simulink model "c172pJSBSim"  (R2026a)
settings: Solver=ode4  StopTime=inf  FixedStep=stepSize_s
undefined symbols (not defined in the file): actuatorDelay_s, plantSampleTime_s, referenceLatitude_deg, referenceLongitude_deg, vehicleParams
settings Model: Creator=GTAR  LastModifiedBy=Edison Altamirano
settings DebuggingCC: ModelReferenceIOMismatchMessage=warning
settings ModelReferenceCC: ModelReferenceNumInstancesAllowed=Single

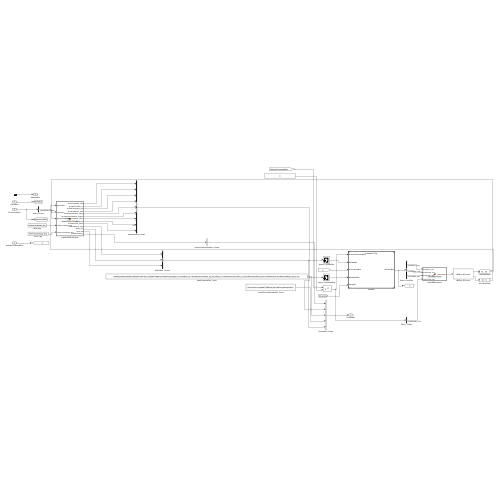
[thumbnail: Simulink's stored preview of the top-level diagram]
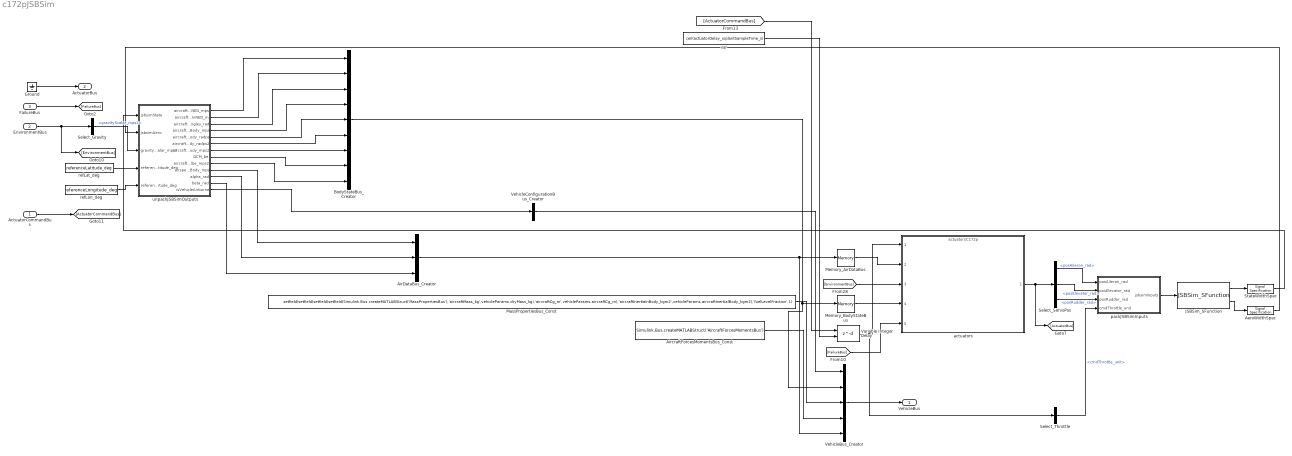
== system c172pJSBSim ==
  ActuatorCommandBus : Inport  OutDataTypeStr=Bus: ActuatorCommandBus
  EnvironmentBus : Inport  Port=2  OutDataTypeStr=Bus: EnvironmentBus
  FailureBus : Inport  Port=3  OutDataTypeStr=Bus: FailureBus
  AeroWidthSpec : SignalSpecification  Dimensions=5
  AirDataBus_Creator : BusCreator  Inputs=3  OutDataTypeStr=Bus: AirDataBus
  AircraftForcesMomentsBus_Const : Constant  Value=Simulink.Bus.createMATLABStruct('AircraftForcesMomentsBus')  OutDataTypeStr=Bus: AircraftForcesMomentsBus
  BodyStateBus_Creator : BusCreator  Inputs=9  OutDataTypeStr=Bus: BodyStateBus
  Ground : Ground
  JSBSim_SFunction : S-Function  FunctionName=JSBSim_SFunction  Parameters='c172p', stepSize_s, 0, '', 'c172pJSBSimInit', 'C:/SITL/AnelloSummer/optimAeroPX4SIL/c172pJSBSim_io.xml'  SFunctionDeploymentMode=off  EnableBusSupport=off
  MassPropertiesBus_Const : Constant  Value=setfield(setfield(setfield(setfield(Simulink.Bus.createMATLABStruct('MassPropertiesBus'),'aircraftMass_kg',vehicleParams.dryMass_kg),'aircraftCg_m',vehicleParams.aircraftCg_m),'aircraftInertiaInBody_kgm2',vehicleParams.aircraftInertialBody_kgm2),'fuelLevelFraction',1)  OutDataTypeStr=Bus: MassPropertiesBus
  Memory_AirDataBus : Memory
  Memory_BodyStateBus : Memory
  Select_Gravity : BusSelector  OutputSignals=EarthEnvironment.gravityScalar_mps2
  Select_ServoPos : BusSelector  OutputSignals=ServosBus.ServosFixedwingPlaneBus.posAileron_rad,ServosBus.ServosFixedwingPlaneBus.posElevator_rad,ServosBus.ServosFixedwingPlaneBus.posRudder_rad
  Select_Throttle : BusSelector  OutputSignals=EngineCommandBus.cmdThrottle_unit
  StateWidthSpec : SignalSpecification  Dimensions=19
  Variable Integer Delay : Delay  DelayLengthSource=Input port
      settings: InputPortMap=u0,p1
  VehicleBus_Creator : BusCreator  Inputs=5  OutDataTypeStr=Bus: VehicleBus
  VehicleConfigurationBus_Creator : BusCreator  Inputs=1  OutDataTypeStr=Bus: VehicleConfigurationBus
  actuators : ModelReference  ModelNameDialog=actuatorsC172p.slx  SimulationMode=Normal  ModelReferenceVersion=5.3
  packJSBSimInputs : MATLAB Function  TreatAsAtomicUnit=on
  refLat_deg : Constant  Value=referenceLatitude_deg
  refLon_deg : Constant  Value=referenceLongitude_deg
  unpackJSBSimOutputs : MATLAB Function  TreatAsAtomicUnit=on
  var : Constant  Value=ceil(actuatorDelay_s/plantSampleTime_s)
  VehicleBus : Outport  OutDataTypeStr=Bus: VehicleBus
  ActuatorBus : Outport  Port=2  OutDataTypeStr=Bus: ActuatorBus
  wires:
  JSBSim_SFunction/2 -> AeroWidthSpec/1
  Ground/1 -> ActuatorBus/1
  unpackJSBSimOutputs/7(aircraftAccelInBody_mps2) -> BodyStateBus_Creator/7
  FailureBus/1 -> [FailureBus]
  Select_Gravity/1 -> unpackJSBSimOutputs/3(gravityScalar_mps2)  "<gravityScalar_mps2>"
  BodyStateBus_Creator/1 -> Memory_BodyStateBus/1, VehicleBus_Creator/2
  ActuatorCommandBus/1 -> [ActuatorCommandBus]
  EnvironmentBus/1 -> [EnvironmentBus], Select_Gravity/1
  refLon_deg/1 -> unpackJSBSimOutputs/5(referenceLongitude_deg)
  refLat_deg/1 -> unpackJSBSimOutputs/4(referenceLatitude_deg)
  unpackJSBSimOutputs/1(aircraftVelInNED_mps) -> BodyStateBus_Creator/1
  [EnvironmentBus] -> actuators/3
  unpackJSBSimOutputs/2(aircraftPosInNED_m) -> BodyStateBus_Creator/2
  [ActuatorCommandBus] -> Variable Integer Delay/1
  unpackJSBSimOutputs/3(aircraftEulerAngles_rad) -> BodyStateBus_Creator/3
  unpackJSBSimOutputs/4(aircraftVelInBody_mps) -> BodyStateBus_Creator/4
  unpackJSBSimOutputs/5(aircraftAngVelInBody_radps) -> BodyStateBus_Creator/5
  unpackJSBSimOutputs/6(aircraftAngAccelInBody_radps2) -> BodyStateBus_Creator/6
  unpackJSBSimOutputs/8(DCM_be) -> BodyStateBus_Creator/8
  unpackJSBSimOutputs/9(aircraftAccelbe_mps2) -> BodyStateBus_Creator/9
  unpackJSBSimOutputs/10(airspeedInBody_mps) -> AirDataBus_Creator/1
  [FailureBus] -> actuators/5
  unpackJSBSimOutputs/11(alpha_rad) -> AirDataBus_Creator/2
  unpackJSBSimOutputs/12(beta_rad) -> AirDataBus_Creator/3
  unpackJSBSimOutputs/13(isVehicleAirborne) -> VehicleConfigurationBus_Creator/1
  var/1 -> Variable Integer Delay/2
  VehicleConfigurationBus_Creator/1 -> VehicleBus_Creator/1
  AirDataBus_Creator/1 -> Memory_AirDataBus/1, VehicleBus_Creator/5
  Memory_AirDataBus/1 -> actuators/2
  MassPropertiesBus_Const/1 -> VehicleBus_Creator/3
  AircraftForcesMomentsBus_Const/1 -> VehicleBus_Creator/4
  Memory_BodyStateBus/1 -> actuators/4
  Variable Integer Delay/1 -> Select_Throttle/1, actuators/1
  VehicleBus_Creator/1 -> VehicleBus/1
  actuators/1 -> [ActuatorBus], Select_ServoPos/1
  Select_ServoPos/1 -> packJSBSimInputs/1(posAileron_rad)  "<posAileron_rad>"
  Select_ServoPos/2 -> packJSBSimInputs/2(posElevator_rad)  "<posElevator_rad>"
  Select_ServoPos/3 -> packJSBSimInputs/3(posRudder_rad)  "<posRudder_rad>"
  AeroWidthSpec/1 -> unpackJSBSimOutputs/2(jsbsimAero)
  Select_Throttle/1 -> packJSBSimInputs/4(cmdThrottle_unit)  "<cmdThrottle_unit>"
  packJSBSimInputs/1(jsbsimInputs) -> JSBSim_SFunction/1
  JSBSim_SFunction/1 -> StateWidthSpec/1
  StateWidthSpec/1 -> unpackJSBSimOutputs/1(jsbsimState)

== matlab function c172pJSBSim/unpackJSBSimOutputs ==
  data: jsbsimState input size=19; aircraftVelInNED_mps output size=3; jsbsimAero input size=5; gravityScalar_mps2 input size=1; referenceLatitude_deg input size=1; referenceLongitude_deg input size=1; aircraftPosInNED_m output size=3; aircraftEulerAngles_rad output size=3; aircraftVelInBody_mps output size=3; aircraftAngVelInBody_radps output size=3; aircraftAngAccelInBody_radps2 output size=3; aircraftAccelInBody_mps2 output size=3; DCM_be output size=[3 3]; aircraftAccelbe_mps2 output size=3; airspeedInBody_mps output size=3; alpha_rad output size=1; beta_rad output size=1; isVehicleAirborne output size=1
function [aircraftVelInNED_mps, aircraftPosInNED_m, aircraftEulerAngles_rad, ...
          aircraftVelInBody_mps, aircraftAngVelInBody_radps, aircraftAngAccelInBody_radps2, ...
          aircraftAccelInBody_mps2, DCM_be, aircraftAccelbe_mps2, ...
          airspeedInBody_mps, alpha_rad, beta_rad, isVehicleAirborne] = ...
          unpackJSBSimOutputs(jsbsimState, jsbsimAero, gravityScalar_mps2, ...
          referenceLatitude_deg, referenceLongitude_deg) %#codegen
% Converts JSBSim_SFunction's raw English-unit "State"/"Aero" output vectors (see
% aircraft/c172p/c172pJSBSim_io.xml for the exact property order this function assumes) into the SI
% BodyStateBus/AirDataBus fields the rest of this SIL expects. See
% PLAN_JSBSIM_SFUNCTION_HYBRID_C172P.md Phase B/C for why each conversion was chosen.
%
% jsbsimState order (19): lat-gc-deg, long-gc-deg, h-sl-ft, phi-rad, theta-rad, psi-rad, u-fps,
%   v-fps, w-fps, p-rad_sec, q-rad_sec, r-rad_sec, udot-ft_sec2, vdot-ft_sec2, wdot-ft_sec2,
%   pdot-rad_sec2, qdot-rad_sec2, rdot-rad_sec2, h-agl-ft
% jsbsimAero order (5): alpha-rad, beta-rad, u-aero-fps, v-aero-fps, w-aero-fps
ft2m = 0.3048;

lat_deg     = jsbsimState(1);
lon_deg     = jsbsimState(2);
h_sl_ft     = jsbsimState(3);
phi_rad     = jsbsimState(4);
theta_rad   = jsbsimState(5);
psi_rad     = jsbsimState(6);
u_fps       = jsbsimState(7);
v_fps       = jsbsimState(8);
w_fps       = jsbsimState(9);
p_radps     = jsbsimState(10);
q_radps     = jsbsimState(11);
r_radps     = jsbsimState(12);
udot_ftps2  = jsbsimState(13);
vdot_ftps2  = jsbsimState(14);
wdot_ftps2  = jsbsimState(15);
pdot_radps2 = jsbsimState(16);
qdot_radps2 = jsbsimState(17);
rdot_radps2 = jsbsimState(18);
h_agl_ft    = jsbsimState(19);

alpha_rad = jsbsimAero(1);
beta_rad  = jsbsimAero(2);
u_aero_fps = jsbsimAero(3);
v_aero_fps = jsbsimAero(4);
w_aero_fps = jsbsimAero(5);

% Nav (NED) -> body DCM, standard 3-2-1 Euler sequence (Aerospace Toolbox, codegen-compatible).
DCM_be = angle2dcm(psi_rad, theta_rad, phi_rad);

% Local flat-Earth tangent-plane position, anchored at this vehicle's own reference lat/lon (same
% point setUpVehicle.m's "c172pJSBSim" case and c172pJSBSimInit.xml use), with zDown absolute
% (-h_sl_ft*ft2m), matching every other vehicle's aircraftInitialPosInNED_m convention (NED origin
% at sea level / height 0, not at the reference altitude). Hand-coded spherical equirectangular
% approximation instead of Aerospace Toolbox's lla2flat -- lla2flat breaks Simulink's MATLAB
% Function block type inference in this MATLAB release (confirmed by isolated reproduction; same
% bug class as the one already documented in optimAeroPX4SIL/CLAUDE.md section 3 for a different
% toolbox call). At the sub-100km scale this SIL operates at, the spherical/WGS84 difference is
% negligible and this SIL has no other geodetic-accuracy requirement anywhere else.
earthRadius_m = 6371000;
dLat_rad = (lat_deg - referenceLatitude_deg) * pi/180;
dLon_rad = (lon_deg - referenceLongitude_deg) * pi/180;
xNorth_m = dLat_rad * earthRadius_m;
yEast_m = dLon_rad * earthRadius_m * cos(referenceLatitude_deg * pi/180);
zDown_m = -h_sl_ft * ft2m;
aircraftPosInNED_m = [xNorth_m; yEast_m; zDown_m];

aircraftVelInBody_mps = [u_fps; v_fps; w_fps] * ft2m;
aircraftVelInNED_mps = DCM_be' * aircraftVelInBody_mps;

aircraftAngVelInBody_radps = [p_radps; q_radps; r_radps];
aircraftAngAccelInBody_radps2 = [pdot_radps2; qdot_radps2; rdot_radps2];

% JSBSim's accelerations/{u,v,w}dot-ft_sec2 are TOTAL body-axis acceleration at the CG (includes
% gravity's contribution via the equations of motion) -- i.e. the same "raw inertial acceleration"
% quantity every other vehicle's plant supplies for this field. `aircraftAccelbe_mps2` must stay
% the RAW acceleration here, NOT specific force: both ins.slx's "Three-axis Inertial Measurement
% Unit" block (aerolibnav) and ANELLO_X3_IMU_Vehicle_fcn_SIL.m already subtract gravity themselves
% (their own g_body/Gb input) to turn raw acceleration into specific force. Subtracting gravity a
% second time here double-counted it, producing a stationary-aircraft accelerometer reading of
% ~2x g (~19.6 m/s^2) instead of ~9.81 m/s^2. Do not re-add a gravity subtraction here.
aircraftAccelInBody_mps2 = [udot_ftps2; vdot_ftps2; wdot_ftps2] * ft2m;
aircraftAccelbe_mps2 = [0; 0; 0]; % TEMPORARY unmistakable test value -- revert after confirming this reaches PX4

aircraftEulerAngles_rad = [phi_rad; theta_rad; psi_rad];

% Airmass-relative body-axis velocity (wind-inclusive) for AirDataBus -- NOT the inertial u/v/w.
airspeedInBody_mps = [u_aero_fps; v_aero_fps; w_aero_fps] * ft2m;

isVehicleAirborne = (h_agl_ft * ft2m) > 0.1;
end

== matlab function c172pJSBSim/packJSBSimInputs ==
  data: posAileron_rad input; jsbsimInputs output; posElevator_rad input; posRudder_rad input; cmdThrottle_unit input
function jsbsimInputs = packJSBSimInputs(posAileron_rad, posElevator_rad, posRudder_rad, cmdThrottle_unit)
%#codegen
% Re-normalizes actuatorsC172p.slx's achieved (rate-limited) surface positions back to JSBSim's
% fcs/*-cmd-norm convention, using the same real deflection limits as setUpActuators.m's "c172p"
% case (sourced from c172p.xml <flight_control> aerosurface_scale ranges: elevator 28 deg,
% aileron 20 deg, rudder 16 deg). Throttle is passed straight through (already 0..1 normalized,
% not rate-limited by actuatorsC172p). Output order matches c172pJSBSim_io.xml <input> order
% exactly: aileron, elevator, rudder, throttle -- do not reorder without updating that file.
maxAilDefl_rad = 20 * pi/180;
maxElevatorDefl_rad = 28 * pi/180;
maxRudderDefl_rad = 16 * pi/180;

aileronCmd_norm = max(min(posAileron_rad / maxAilDefl_rad, 1), -1);
elevatorCmd_norm = max(min(posElevator_rad / maxElevatorDefl_rad, 1), -1);
rudderCmd_norm = max(min(posRudder_rad / maxRudderDefl_rad, 1), -1);
throttleCmd_norm = max(min(cmdThrottle_unit, 1), 0);

jsbsimInputs = [aileronCmd_norm; elevatorCmd_norm; rudderCmd_norm; throttleCmd_norm];
end
